simulink model "Approx_Multiplier_M1_AMA1"  (R2021a)
settings: Solver=VariableStepAuto  StartTime=0.0  StopTime=0.01  RelTol=1e-3
(part 2 of 3)

== system Approx_Multiplier_M1_AMA1/Full Adder33 ==
  A : Inport
  B : Inport  Port=2
  Cin : Inport  Port=3
  Half Adder : Subsystem
  Half Adder1 : Subsystem
  Logical Operator : Logic  Operator=OR  AllPortsSameDT=off  OutDataTypeStr=boolean
  Sum : Outport
  Carry : Outport  Port=2
  wires:
  Cin/1 -> Half Adder1/1(In)
  Half Adder1/2(Cout) -> Logical Operator/1
  Half Adder/1(Sum) -> Half Adder1/2(Cin)
  Half Adder1/1(Sum) -> Sum/1
  Half Adder/2(Cout) -> Logical Operator/2
  A/1 -> Half Adder/1(In)
  B/1 -> Half Adder/2(Cin)
  Logical Operator/1 -> Carry/1

== system Approx_Multiplier_M1_AMA1/Full Adder34 ==
  A : Inport
  B : Inport  Port=2
  Cin : Inport  Port=3
  Half Adder : Subsystem
  Half Adder1 : Subsystem
  Logical Operator : Logic  Operator=OR  AllPortsSameDT=off  OutDataTypeStr=boolean
  Sum : Outport
  Carry : Outport  Port=2
  wires:
  Cin/1 -> Half Adder1/1(In)
  Half Adder1/2(Cout) -> Logical Operator/1
  Half Adder/1(Sum) -> Half Adder1/2(Cin)
  Half Adder1/1(Sum) -> Sum/1
  Half Adder/2(Cout) -> Logical Operator/2
  A/1 -> Half Adder/1(In)
  B/1 -> Half Adder/2(Cin)
  Logical Operator/1 -> Carry/1

== system Approx_Multiplier_M1_AMA1/Full Adder36 ==
  A : Inport
  B : Inport  Port=2
  Cin : Inport  Port=3
  Half Adder : Subsystem
  Half Adder1 : Subsystem
  Logical Operator : Logic  Operator=OR  AllPortsSameDT=off  OutDataTypeStr=boolean
  Sum : Outport
  Carry : Outport  Port=2
  wires:
  Cin/1 -> Half Adder1/1(In)
  Half Adder1/2(Cout) -> Logical Operator/1
  Half Adder/1(Sum) -> Half Adder1/2(Cin)
  Half Adder1/1(Sum) -> Sum/1
  Half Adder/2(Cout) -> Logical Operator/2
  A/1 -> Half Adder/1(In)
  B/1 -> Half Adder/2(Cin)
  Logical Operator/1 -> Carry/1

== system Approx_Multiplier_M1_AMA1/Full Adder37 ==
  A : Inport
  B : Inport  Port=2
  Cin : Inport  Port=3
  Half Adder : Subsystem
  Half Adder1 : Subsystem
  Logical Operator : Logic  Operator=OR  AllPortsSameDT=off  OutDataTypeStr=boolean
  Sum : Outport
  Carry : Outport  Port=2
  wires:
  Cin/1 -> Half Adder1/1(In)
  Half Adder1/2(Cout) -> Logical Operator/1
  Half Adder/1(Sum) -> Half Adder1/2(Cin)
  Half Adder1/1(Sum) -> Sum/1
  Half Adder/2(Cout) -> Logical Operator/2
  A/1 -> Half Adder/1(In)
  B/1 -> Half Adder/2(Cin)
  Logical Operator/1 -> Carry/1

== system Approx_Multiplier_M1_AMA1/Full Adder38 ==
  A : Inport
  B : Inport  Port=2
  Cin : Inport  Port=3
  Half Adder : Subsystem
  Half Adder1 : Subsystem
  Logical Operator : Logic  Operator=OR  AllPortsSameDT=off  OutDataTypeStr=boolean
  Sum : Outport
  Carry : Outport  Port=2
  wires:
  Cin/1 -> Half Adder1/1(In)
  Half Adder1/2(Cout) -> Logical Operator/1
  Half Adder/1(Sum) -> Half Adder1/2(Cin)
  Half Adder1/1(Sum) -> Sum/1
  Half Adder/2(Cout) -> Logical Operator/2
  A/1 -> Half Adder/1(In)
  B/1 -> Half Adder/2(Cin)
  Logical Operator/1 -> Carry/1

== system Approx_Multiplier_M1_AMA1/Full Adder39 ==
  A : Inport
  B : Inport  Port=2
  Cin : Inport  Port=3
  Half Adder : Subsystem
  Half Adder1 : Subsystem
  Logical Operator : Logic  Operator=OR  AllPortsSameDT=off  OutDataTypeStr=boolean
  Sum : Outport
  Carry : Outport  Port=2
  wires:
  Cin/1 -> Half Adder1/1(In)
  Half Adder1/2(Cout) -> Logical Operator/1
  Half Adder/1(Sum) -> Half Adder1/2(Cin)
  Half Adder1/1(Sum) -> Sum/1
  Half Adder/2(Cout) -> Logical Operator/2
  A/1 -> Half Adder/1(In)
  B/1 -> Half Adder/2(Cin)
  Logical Operator/1 -> Carry/1

== system Approx_Multiplier_M1_AMA1/Full Adder40 ==
  A : Inport
  B : Inport  Port=2
  Cin : Inport  Port=3
  Half Adder : Subsystem
  Half Adder1 : Subsystem
  Logical Operator : Logic  Operator=OR  AllPortsSameDT=off  OutDataTypeStr=boolean
  Sum : Outport
  Carry : Outport  Port=2
  wires:
  Cin/1 -> Half Adder1/1(In)
  Half Adder1/2(Cout) -> Logical Operator/1
  Half Adder/1(Sum) -> Half Adder1/2(Cin)
  Half Adder1/1(Sum) -> Sum/1
  Half Adder/2(Cout) -> Logical Operator/2
  A/1 -> Half Adder/1(In)
  B/1 -> Half Adder/2(Cin)
  Logical Operator/1 -> Carry/1

== system Approx_Multiplier_M1_AMA1/Full Adder41 ==
  A : Inport
  B : Inport  Port=2
  Cin : Inport  Port=3
  Half Adder : Subsystem
  Half Adder1 : Subsystem
  Logical Operator : Logic  Operator=OR  AllPortsSameDT=off  OutDataTypeStr=boolean
  Sum : Outport
  Carry : Outport  Port=2
  wires:
  Cin/1 -> Half Adder1/1(In)
  Half Adder1/2(Cout) -> Logical Operator/1
  Half Adder/1(Sum) -> Half Adder1/2(Cin)
  Half Adder1/1(Sum) -> Sum/1
  Half Adder/2(Cout) -> Logical Operator/2
  A/1 -> Half Adder/1(In)
  B/1 -> Half Adder/2(Cin)
  Logical Operator/1 -> Carry/1

== system Approx_Multiplier_M1_AMA1/Full Adder42 ==
  A : Inport
  B : Inport  Port=2
  Cin : Inport  Port=3
  Half Adder : Subsystem
  Half Adder1 : Subsystem
  Logical Operator : Logic  Operator=OR  AllPortsSameDT=off  OutDataTypeStr=boolean
  Sum : Outport
  Carry : Outport  Port=2
  wires:
  Cin/1 -> Half Adder1/1(In)
  Half Adder1/2(Cout) -> Logical Operator/1
  Half Adder/1(Sum) -> Half Adder1/2(Cin)
  Half Adder1/1(Sum) -> Sum/1
  Half Adder/2(Cout) -> Logical Operator/2
  A/1 -> Half Adder/1(In)
  B/1 -> Half Adder/2(Cin)
  Logical Operator/1 -> Carry/1

== system Approx_Multiplier_M1_AMA1/Full Adder43 ==
  A : Inport
  B : Inport  Port=2
  Cin : Inport  Port=3
  Half Adder : Subsystem
  Half Adder1 : Subsystem
  Logical Operator : Logic  Operator=OR  AllPortsSameDT=off  OutDataTypeStr=boolean
  Sum : Outport
  Carry : Outport  Port=2
  wires:
  Cin/1 -> Half Adder1/1(In)
  Half Adder1/2(Cout) -> Logical Operator/1
  Half Adder/1(Sum) -> Half Adder1/2(Cin)
  Half Adder1/1(Sum) -> Sum/1
  Half Adder/2(Cout) -> Logical Operator/2
  A/1 -> Half Adder/1(In)
  B/1 -> Half Adder/2(Cin)
  Logical Operator/1 -> Carry/1

== system Approx_Multiplier_M1_AMA1/Full Adder44 ==
  A : Inport
  B : Inport  Port=2
  Cin : Inport  Port=3
  Half Adder : Subsystem
  Half Adder1 : Subsystem
  Logical Operator : Logic  Operator=OR  AllPortsSameDT=off  OutDataTypeStr=boolean
  Sum : Outport
  Carry : Outport  Port=2
  wires:
  Cin/1 -> Half Adder1/1(In)
  Half Adder1/2(Cout) -> Logical Operator/1
  Half Adder/1(Sum) -> Half Adder1/2(Cin)
  Half Adder1/1(Sum) -> Sum/1
  Half Adder/2(Cout) -> Logical Operator/2
  A/1 -> Half Adder/1(In)
  B/1 -> Half Adder/2(Cin)
  Logical Operator/1 -> Carry/1

== system Approx_Multiplier_M1_AMA1/Full Adder45 ==
  A : Inport
  B : Inport  Port=2
  Cin : Inport  Port=3
  Half Adder : Subsystem
  Half Adder1 : Subsystem
  Logical Operator : Logic  Operator=OR  AllPortsSameDT=off  OutDataTypeStr=boolean
  Sum : Outport
  Carry : Outport  Port=2
  wires:
  Cin/1 -> Half Adder1/1(In)
  Half Adder1/2(Cout) -> Logical Operator/1
  Half Adder/1(Sum) -> Half Adder1/2(Cin)
  Half Adder1/1(Sum) -> Sum/1
  Half Adder/2(Cout) -> Logical Operator/2
  A/1 -> Half Adder/1(In)
  B/1 -> Half Adder/2(Cin)
  Logical Operator/1 -> Carry/1

== system Approx_Multiplier_M1_AMA1/Full Adder46 ==
  A : Inport
  B : Inport  Port=2
  Cin : Inport  Port=3
  Half Adder : Subsystem
  Half Adder1 : Subsystem
  Logical Operator : Logic  Operator=OR  AllPortsSameDT=off  OutDataTypeStr=boolean
  Sum : Outport
  Carry : Outport  Port=2
  wires:
  Cin/1 -> Half Adder1/1(In)
  Half Adder1/2(Cout) -> Logical Operator/1
  Half Adder/1(Sum) -> Half Adder1/2(Cin)
  Half Adder1/1(Sum) -> Sum/1
  Half Adder/2(Cout) -> Logical Operator/2
  A/1 -> Half Adder/1(In)
  B/1 -> Half Adder/2(Cin)
  Logical Operator/1 -> Carry/1

== system Approx_Multiplier_M1_AMA1/Full Adder47 ==
  A : Inport
  B : Inport  Port=2
  Cin : Inport  Port=3
  Half Adder : Subsystem
  Half Adder1 : Subsystem
  Logical Operator : Logic  Operator=OR  AllPortsSameDT=off  OutDataTypeStr=boolean
  Sum : Outport
  Carry : Outport  Port=2
  wires:
  Cin/1 -> Half Adder1/1(In)
  Half Adder1/2(Cout) -> Logical Operator/1
  Half Adder/1(Sum) -> Half Adder1/2(Cin)
  Half Adder1/1(Sum) -> Sum/1
  Half Adder/2(Cout) -> Logical Operator/2
  A/1 -> Half Adder/1(In)
  B/1 -> Half Adder/2(Cin)
  Logical Operator/1 -> Carry/1

== system Approx_Multiplier_M1_AMA1/Full Adder48 ==
  A : Inport
  B : Inport  Port=2
  Cin : Inport  Port=3
  Half Adder : Subsystem
  Half Adder1 : Subsystem
  Logical Operator : Logic  Operator=OR  AllPortsSameDT=off  OutDataTypeStr=boolean
  Sum : Outport
  Carry : Outport  Port=2
  wires:
  Cin/1 -> Half Adder1/1(In)
  Half Adder1/2(Cout) -> Logical Operator/1
  Half Adder/1(Sum) -> Half Adder1/2(Cin)
  Half Adder1/1(Sum) -> Sum/1
  Half Adder/2(Cout) -> Logical Operator/2
  A/1 -> Half Adder/1(In)
  B/1 -> Half Adder/2(Cin)
  Logical Operator/1 -> Carry/1

== system Approx_Multiplier_M1_AMA1/Full Adder6 ==
  A : Inport
  B : Inport  Port=2
  Cin : Inport  Port=3
  Half Adder : Subsystem
  Half Adder1 : Subsystem
  Logical Operator : Logic  Operator=OR  AllPortsSameDT=off  OutDataTypeStr=boolean
  Sum : Outport
  Carry : Outport  Port=2
  wires:
  Cin/1 -> Half Adder1/1(In)
  Half Adder1/2(Cout) -> Logical Operator/1
  Half Adder/1(Sum) -> Half Adder1/2(Cin)
  Half Adder1/1(Sum) -> Sum/1
  Half Adder/2(Cout) -> Logical Operator/2
  A/1 -> Half Adder/1(In)
  B/1 -> Half Adder/2(Cin)
  Logical Operator/1 -> Carry/1

== system Approx_Multiplier_M1_AMA1/Half Adder10 ==
  A7B2 : Inport
  Cin : Inport  Port=2
  Logical Operator : Logic  Operator=XOR  AllPortsSameDT=off  OutDataTypeStr=boolean
  Logical Operator1 : Logic  AllPortsSameDT=off  OutDataTypeStr=boolean
  Sum : Outport
  Cout : Outport  Port=2
  wires:
  A7B2/1 -> Logical Operator1/1, Logical Operator/1
  Cin/1 -> Logical Operator/2, Logical Operator1/2
  Logical Operator/1 -> Sum/1
  Logical Operator1/1 -> Cout/1

== system Approx_Multiplier_M1_AMA1/Half Adder11 ==
  A7B2 : Inport
  Cin : Inport  Port=2
  Logical Operator : Logic  Operator=XOR  AllPortsSameDT=off  OutDataTypeStr=boolean
  Logical Operator1 : Logic  AllPortsSameDT=off  OutDataTypeStr=boolean
  Sum : Outport
  Cout : Outport  Port=2
  wires:
  A7B2/1 -> Logical Operator1/1, Logical Operator/1
  Cin/1 -> Logical Operator/2, Logical Operator1/2
  Logical Operator/1 -> Sum/1
  Logical Operator1/1 -> Cout/1

== system Approx_Multiplier_M1_AMA1/Half Adder12 ==
  A7B2 : Inport
  Cin : Inport  Port=2
  Logical Operator : Logic  Operator=XOR  AllPortsSameDT=off  OutDataTypeStr=boolean
  Logical Operator1 : Logic  AllPortsSameDT=off  OutDataTypeStr=boolean
  Sum : Outport
  Cout : Outport  Port=2
  wires:
  A7B2/1 -> Logical Operator1/1, Logical Operator/1
  Cin/1 -> Logical Operator/2, Logical Operator1/2
  Logical Operator/1 -> Sum/1
  Logical Operator1/1 -> Cout/1

== system Approx_Multiplier_M1_AMA1/Half Adder13 ==
  A7B2 : Inport
  Cin : Inport  Port=2
  Logical Operator : Logic  Operator=XOR  AllPortsSameDT=off  OutDataTypeStr=boolean
  Logical Operator1 : Logic  AllPortsSameDT=off  OutDataTypeStr=boolean
  Sum : Outport
  Cout : Outport  Port=2
  wires:
  A7B2/1 -> Logical Operator1/1, Logical Operator/1
  Cin/1 -> Logical Operator/2, Logical Operator1/2
  Logical Operator/1 -> Sum/1
  Logical Operator1/1 -> Cout/1

== system Approx_Multiplier_M1_AMA1/Half Adder7 ==
  Cin : Inport
  Cin1 : Inport  Port=2
  Logical Operator : Logic  Operator=XOR  AllPortsSameDT=off  OutDataTypeStr=boolean
  Logical Operator1 : Logic  AllPortsSameDT=off  OutDataTypeStr=boolean
  Sum : Outport
  Cout : Outport  Port=2
  wires:
  Cin/1 -> Logical Operator1/2, Logical Operator/2
  Logical Operator/1 -> Sum/1
  Logical Operator1/1 -> Cout/1
  Cin1/1 -> Logical Operator1/1, Logical Operator/1

== system Approx_Multiplier_M1_AMA1/Half Adder8 ==
  A7B2 : Inport
  Cin : Inport  Port=2
  Logical Operator : Logic  Operator=XOR  AllPortsSameDT=off  OutDataTypeStr=boolean
  Logical Operator1 : Logic  AllPortsSameDT=off  OutDataTypeStr=boolean
  Sum : Outport
  Cout : Outport  Port=2
  wires:
  A7B2/1 -> Logical Operator1/1, Logical Operator/1
  Cin/1 -> Logical Operator/2, Logical Operator1/2
  Logical Operator/1 -> Sum/1
  Logical Operator1/1 -> Cout/1

== system Approx_Multiplier_M1_AMA1/Half Adder9 ==
  A7B2 : Inport
  Cin : Inport  Port=2
  Logical Operator : Logic  Operator=XOR  AllPortsSameDT=off  OutDataTypeStr=boolean
  Logical Operator1 : Logic  AllPortsSameDT=off  OutDataTypeStr=boolean
  Sum : Outport
  Cout : Outport  Port=2
  wires:
  A7B2/1 -> Logical Operator1/1, Logical Operator/1
  Cin/1 -> Logical Operator/2, Logical Operator1/2
  Logical Operator/1 -> Sum/1
  Logical Operator1/1 -> Cout/1

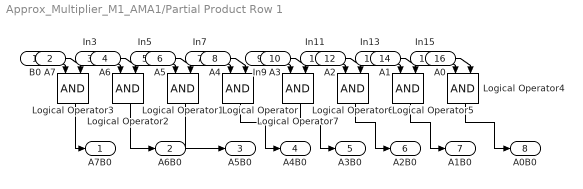
== system Approx_Multiplier_M1_AMA1/Partial Product Row 1 ==
  B0 : Inport
  A7 : Inport  Port=2
  In3 : Inport  Port=3
  A6 : Inport  Port=4
  In5 : Inport  Port=5
  A5 : Inport  Port=6
  In7 : Inport  Port=7
  A4 : Inport  Port=8
  In9 : Inport  Port=9
  A3 : Inport  Port=10
  In11 : Inport  Port=11
  A2 : Inport  Port=12
  In13 : Inport  Port=13
  A1 : Inport  Port=14
  In15 : Inport  Port=15
  A0 : Inport  Port=16
  Logical Operator{,1..7} (8 alike) : Logic  AllPortsSameDT=off  OutDataTypeStr=boolean
  A7B0 : Outport
  A6B0 : Outport  Port=2
  A5B0 : Outport  Port=3
  A4B0 : Outport  Port=4
  A3B0 : Outport  Port=5
  A2B0 : Outport  Port=6
  A1B0 : Outport  Port=7
  A0B0 : Outport  Port=8
  wires:
  Logical Operator7/1 -> A3B0/1
  Logical Operator4/1 -> A0B0/1
  A4/1 -> Logical Operator/2
  Logical Operator/1 -> A4B0/1
  Logical Operator1/1 -> A5B0/1
  A7/1 -> Logical Operator3/2
  In11/1 -> Logical Operator6/1
  In5/1 -> Logical Operator1/1
  A5/1 -> Logical Operator1/2
  In7/1 -> Logical Operator/1
  A6/1 -> Logical Operator2/2
  B0/1 -> Logical Operator3/1
  A2/1 -> Logical Operator6/2
  Logical Operator3/1 -> A7B0/1
  In3/1 -> Logical Operator2/1
  Logical Operator2/1 -> A6B0/1
  In13/1 -> Logical Operator5/1
  A1/1 -> Logical Operator5/2
  Logical Operator5/1 -> A1B0/1
  Logical Operator6/1 -> A2B0/1
  In9/1 -> Logical Operator7/1
  A3/1 -> Logical Operator7/2
  In15/1 -> Logical Operator4/1
  A0/1 -> Logical Operator4/2

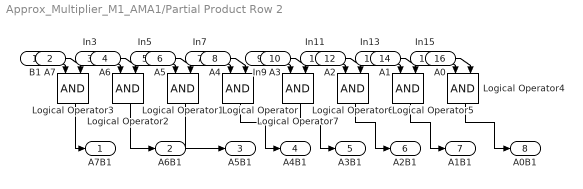
== system Approx_Multiplier_M1_AMA1/Partial Product Row 2 ==
  B1 : Inport
  A7 : Inport  Port=2
  In3 : Inport  Port=3
  A6 : Inport  Port=4
  In5 : Inport  Port=5
  A5 : Inport  Port=6
  In7 : Inport  Port=7
  A4 : Inport  Port=8
  In9 : Inport  Port=9
  A3 : Inport  Port=10
  In11 : Inport  Port=11
  A2 : Inport  Port=12
  In13 : Inport  Port=13
  A1 : Inport  Port=14
  In15 : Inport  Port=15
  A0 : Inport  Port=16
  Logical Operator{,1..7} (8 alike) : Logic  AllPortsSameDT=off  OutDataTypeStr=boolean
  A7B1 : Outport
  A6B1 : Outport  Port=2
  A5B1 : Outport  Port=3
  A4B1 : Outport  Port=4
  A3B1 : Outport  Port=5
  A2B1 : Outport  Port=6
  A1B1 : Outport  Port=7
  A0B1 : Outport  Port=8
  wires:
  Logical Operator7/1 -> A3B1/1
  Logical Operator4/1 -> A0B1/1
  A4/1 -> Logical Operator/2
  Logical Operator/1 -> A4B1/1
  Logical Operator1/1 -> A5B1/1
  A7/1 -> Logical Operator3/2
  In11/1 -> Logical Operator6/1
  In5/1 -> Logical Operator1/1
  A5/1 -> Logical Operator1/2
  In7/1 -> Logical Operator/1
  A6/1 -> Logical Operator2/2
  B1/1 -> Logical Operator3/1
  A2/1 -> Logical Operator6/2
  Logical Operator3/1 -> A7B1/1
  In3/1 -> Logical Operator2/1
  Logical Operator2/1 -> A6B1/1
  In13/1 -> Logical Operator5/1
  A1/1 -> Logical Operator5/2
  Logical Operator5/1 -> A1B1/1
  Logical Operator6/1 -> A2B1/1
  In9/1 -> Logical Operator7/1
  A3/1 -> Logical Operator7/2
  In15/1 -> Logical Operator4/1
  A0/1 -> Logical Operator4/2

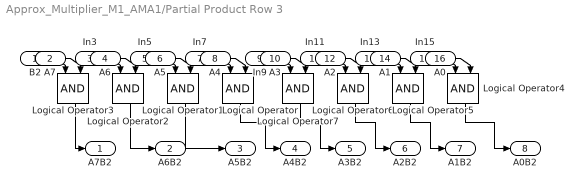
== system Approx_Multiplier_M1_AMA1/Partial Product Row 3 ==
  B2 : Inport
  A7 : Inport  Port=2
  In3 : Inport  Port=3
  A6 : Inport  Port=4
  In5 : Inport  Port=5
  A5 : Inport  Port=6
  In7 : Inport  Port=7
  A4 : Inport  Port=8
  In9 : Inport  Port=9
  A3 : Inport  Port=10
  In11 : Inport  Port=11
  A2 : Inport  Port=12
  In13 : Inport  Port=13
  A1 : Inport  Port=14
  In15 : Inport  Port=15
  A0 : Inport  Port=16
  Logical Operator{,1..7} (8 alike) : Logic  AllPortsSameDT=off  OutDataTypeStr=boolean
  A7B2 : Outport
  A6B2 : Outport  Port=2
  A5B2 : Outport  Port=3
  A4B2 : Outport  Port=4
  A3B2 : Outport  Port=5
  A2B2 : Outport  Port=6
  A1B2 : Outport  Port=7
  A0B2 : Outport  Port=8
  wires:
  Logical Operator7/1 -> A3B2/1
  Logical Operator4/1 -> A0B2/1
  A4/1 -> Logical Operator/2
  Logical Operator/1 -> A4B2/1
  Logical Operator1/1 -> A5B2/1
  A7/1 -> Logical Operator3/2
  In11/1 -> Logical Operator6/1
  In5/1 -> Logical Operator1/1
  A5/1 -> Logical Operator1/2
  In7/1 -> Logical Operator/1
  A6/1 -> Logical Operator2/2
  B2/1 -> Logical Operator3/1
  A2/1 -> Logical Operator6/2
  Logical Operator3/1 -> A7B2/1
  In3/1 -> Logical Operator2/1
  Logical Operator2/1 -> A6B2/1
  In13/1 -> Logical Operator5/1
  A1/1 -> Logical Operator5/2
  Logical Operator5/1 -> A1B2/1
  Logical Operator6/1 -> A2B2/1
  In9/1 -> Logical Operator7/1
  A3/1 -> Logical Operator7/2
  In15/1 -> Logical Operator4/1
  A0/1 -> Logical Operator4/2

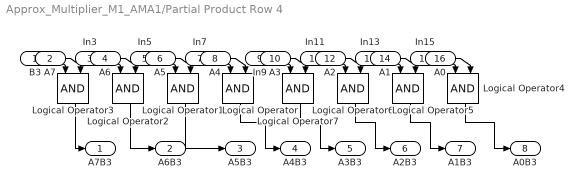
== system Approx_Multiplier_M1_AMA1/Partial Product Row 4 ==
  B3 : Inport
  A7 : Inport  Port=2
  In3 : Inport  Port=3
  A6 : Inport  Port=4
  In5 : Inport  Port=5
  A5 : Inport  Port=6
  In7 : Inport  Port=7
  A4 : Inport  Port=8
  In9 : Inport  Port=9
  A3 : Inport  Port=10
  In11 : Inport  Port=11
  A2 : Inport  Port=12
  In13 : Inport  Port=13
  A1 : Inport  Port=14
  In15 : Inport  Port=15
  A0 : Inport  Port=16
  Logical Operator{,1..7} (8 alike) : Logic  AllPortsSameDT=off  OutDataTypeStr=boolean
  A7B3 : Outport
  A6B3 : Outport  Port=2
  A5B3 : Outport  Port=3
  A4B3 : Outport  Port=4
  A3B3 : Outport  Port=5
  A2B3 : Outport  Port=6
  A1B3 : Outport  Port=7
  A0B3 : Outport  Port=8
  wires:
  Logical Operator7/1 -> A3B3/1
  Logical Operator4/1 -> A0B3/1
  A4/1 -> Logical Operator/2
  Logical Operator/1 -> A4B3/1
  Logical Operator1/1 -> A5B3/1
  A7/1 -> Logical Operator3/2
  In11/1 -> Logical Operator6/1
  In5/1 -> Logical Operator1/1
  A5/1 -> Logical Operator1/2
  In7/1 -> Logical Operator/1
  A6/1 -> Logical Operator2/2
  B3/1 -> Logical Operator3/1
  A2/1 -> Logical Operator6/2
  Logical Operator3/1 -> A7B3/1
  In3/1 -> Logical Operator2/1
  Logical Operator2/1 -> A6B3/1
  In13/1 -> Logical Operator5/1
  A1/1 -> Logical Operator5/2
  Logical Operator5/1 -> A1B3/1
  Logical Operator6/1 -> A2B3/1
  In9/1 -> Logical Operator7/1
  A3/1 -> Logical Operator7/2
  In15/1 -> Logical Operator4/1
  A0/1 -> Logical Operator4/2

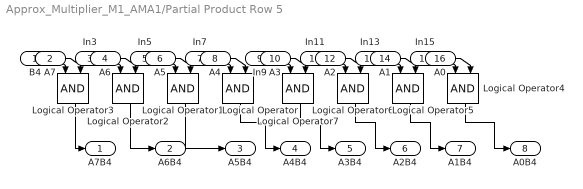
== system Approx_Multiplier_M1_AMA1/Partial Product Row 5 ==
  B4 : Inport
  A7 : Inport  Port=2
  In3 : Inport  Port=3
  A6 : Inport  Port=4
  In5 : Inport  Port=5
  A5 : Inport  Port=6
  In7 : Inport  Port=7
  A4 : Inport  Port=8
  In9 : Inport  Port=9
  A3 : Inport  Port=10
  In11 : Inport  Port=11
  A2 : Inport  Port=12
  In13 : Inport  Port=13
  A1 : Inport  Port=14
  In15 : Inport  Port=15
  A0 : Inport  Port=16
  Logical Operator{,1..7} (8 alike) : Logic  AllPortsSameDT=off  OutDataTypeStr=boolean
  A7B4 : Outport
  A6B4 : Outport  Port=2
  A5B4 : Outport  Port=3
  A4B4 : Outport  Port=4
  A3B4 : Outport  Port=5
  A2B4 : Outport  Port=6
  A1B4 : Outport  Port=7
  A0B4 : Outport  Port=8
  wires:
  Logical Operator7/1 -> A3B4/1
  Logical Operator4/1 -> A0B4/1
  A4/1 -> Logical Operator/2
  Logical Operator/1 -> A4B4/1
  Logical Operator1/1 -> A5B4/1
  A7/1 -> Logical Operator3/2
  In11/1 -> Logical Operator6/1
  In5/1 -> Logical Operator1/1
  A5/1 -> Logical Operator1/2
  In7/1 -> Logical Operator/1
  A6/1 -> Logical Operator2/2
  B4/1 -> Logical Operator3/1
  A2/1 -> Logical Operator6/2
  Logical Operator3/1 -> A7B4/1
  In3/1 -> Logical Operator2/1
  Logical Operator2/1 -> A6B4/1
  In13/1 -> Logical Operator5/1
  A1/1 -> Logical Operator5/2
  Logical Operator5/1 -> A1B4/1
  Logical Operator6/1 -> A2B4/1
  In9/1 -> Logical Operator7/1
  A3/1 -> Logical Operator7/2
  In15/1 -> Logical Operator4/1
  A0/1 -> Logical Operator4/2

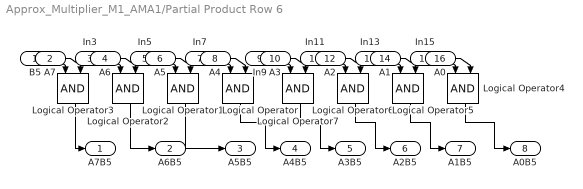
== system Approx_Multiplier_M1_AMA1/Partial Product Row 6 ==
  B5 : Inport
  A7 : Inport  Port=2
  In3 : Inport  Port=3
  A6 : Inport  Port=4
  In5 : Inport  Port=5
  A5 : Inport  Port=6
  In7 : Inport  Port=7
  A4 : Inport  Port=8
  In9 : Inport  Port=9
  A3 : Inport  Port=10
  In11 : Inport  Port=11
  A2 : Inport  Port=12
  In13 : Inport  Port=13
  A1 : Inport  Port=14
  In15 : Inport  Port=15
  A0 : Inport  Port=16
  Logical Operator{,1..7} (8 alike) : Logic  AllPortsSameDT=off  OutDataTypeStr=boolean
  A7B5 : Outport
  A6B5 : Outport  Port=2
  A5B5 : Outport  Port=3
  A4B5 : Outport  Port=4
  A3B5 : Outport  Port=5
  A2B5 : Outport  Port=6
  A1B5 : Outport  Port=7
  A0B5 : Outport  Port=8
  wires:
  Logical Operator7/1 -> A3B5/1
  Logical Operator4/1 -> A0B5/1
  A4/1 -> Logical Operator/2
  Logical Operator/1 -> A4B5/1
  Logical Operator1/1 -> A5B5/1
  A7/1 -> Logical Operator3/2
  In11/1 -> Logical Operator6/1
  In5/1 -> Logical Operator1/1
  A5/1 -> Logical Operator1/2
  In7/1 -> Logical Operator/1
  A6/1 -> Logical Operator2/2
  B5/1 -> Logical Operator3/1
  A2/1 -> Logical Operator6/2
  Logical Operator3/1 -> A7B5/1
  In3/1 -> Logical Operator2/1
  Logical Operator2/1 -> A6B5/1
  In13/1 -> Logical Operator5/1
  A1/1 -> Logical Operator5/2
  Logical Operator5/1 -> A1B5/1
  Logical Operator6/1 -> A2B5/1
  In9/1 -> Logical Operator7/1
  A3/1 -> Logical Operator7/2
  In15/1 -> Logical Operator4/1
  A0/1 -> Logical Operator4/2

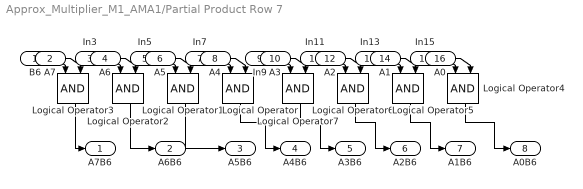
== system Approx_Multiplier_M1_AMA1/Partial Product Row 7 ==
  B6 : Inport
  A7 : Inport  Port=2
  In3 : Inport  Port=3
  A6 : Inport  Port=4
  In5 : Inport  Port=5
  A5 : Inport  Port=6
  In7 : Inport  Port=7
  A4 : Inport  Port=8
  In9 : Inport  Port=9
  A3 : Inport  Port=10
  In11 : Inport  Port=11
  A2 : Inport  Port=12
  In13 : Inport  Port=13
  A1 : Inport  Port=14
  In15 : Inport  Port=15
  A0 : Inport  Port=16
  Logical Operator{,1..7} (8 alike) : Logic  AllPortsSameDT=off  OutDataTypeStr=boolean
  A7B6 : Outport
  A6B6 : Outport  Port=2
  A5B6 : Outport  Port=3
  A4B6 : Outport  Port=4
  A3B6 : Outport  Port=5
  A2B6 : Outport  Port=6
  A1B6 : Outport  Port=7
  A0B6 : Outport  Port=8
  wires:
  Logical Operator7/1 -> A3B6/1
  Logical Operator4/1 -> A0B6/1
  A4/1 -> Logical Operator/2
  Logical Operator/1 -> A4B6/1
  Logical Operator1/1 -> A5B6/1
  A7/1 -> Logical Operator3/2
  In11/1 -> Logical Operator6/1
  In5/1 -> Logical Operator1/1
  A5/1 -> Logical Operator1/2
  In7/1 -> Logical Operator/1
  A6/1 -> Logical Operator2/2
  B6/1 -> Logical Operator3/1
  A2/1 -> Logical Operator6/2
  Logical Operator3/1 -> A7B6/1
  In3/1 -> Logical Operator2/1
  Logical Operator2/1 -> A6B6/1
  In13/1 -> Logical Operator5/1
  A1/1 -> Logical Operator5/2
  Logical Operator5/1 -> A1B6/1
  Logical Operator6/1 -> A2B6/1
  In9/1 -> Logical Operator7/1
  A3/1 -> Logical Operator7/2
  In15/1 -> Logical Operator4/1
  A0/1 -> Logical Operator4/2

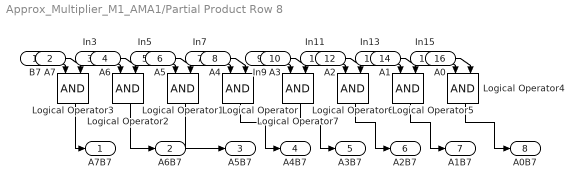
== system Approx_Multiplier_M1_AMA1/Partial Product Row 8 ==
  B7 : Inport
  A7 : Inport  Port=2
  In3 : Inport  Port=3
  A6 : Inport  Port=4
  In5 : Inport  Port=5
  A5 : Inport  Port=6
  In7 : Inport  Port=7
  A4 : Inport  Port=8
  In9 : Inport  Port=9
  A3 : Inport  Port=10
  In11 : Inport  Port=11
  A2 : Inport  Port=12
  In13 : Inport  Port=13
  A1 : Inport  Port=14
  In15 : Inport  Port=15
  A0 : Inport  Port=16
  Logical Operator{,1..7} (8 alike) : Logic  AllPortsSameDT=off  OutDataTypeStr=boolean
  A7B7 : Outport
  A6B7 : Outport  Port=2
  A5B7 : Outport  Port=3
  A4B7 : Outport  Port=4
  A3B7 : Outport  Port=5
  A2B7 : Outport  Port=6
  A1B7 : Outport  Port=7
  A0B7 : Outport  Port=8
  wires:
  Logical Operator7/1 -> A3B7/1
  Logical Operator4/1 -> A0B7/1
  A4/1 -> Logical Operator/2
  Logical Operator/1 -> A4B7/1
  Logical Operator1/1 -> A5B7/1
  A7/1 -> Logical Operator3/2
  In11/1 -> Logical Operator6/1
  In5/1 -> Logical Operator1/1
  A5/1 -> Logical Operator1/2
  In7/1 -> Logical Operator/1
  A6/1 -> Logical Operator2/2
  B7/1 -> Logical Operator3/1
  A2/1 -> Logical Operator6/2
  Logical Operator3/1 -> A7B7/1
  In3/1 -> Logical Operator2/1
  Logical Operator2/1 -> A6B7/1
  In13/1 -> Logical Operator5/1
  A1/1 -> Logical Operator5/2
  Logical Operator5/1 -> A1B7/1
  Logical Operator6/1 -> A2B7/1
  In9/1 -> Logical Operator7/1
  A3/1 -> Logical Operator7/2
  In15/1 -> Logical Operator4/1
  A0/1 -> Logical Operator4/2

== system Approx_Multiplier_M1_AMA1/Full Adder12/Half Adder ==
  In : Inport
  Cin : Inport  Port=2
  Logical Operator : Logic  Operator=XOR  AllPortsSameDT=off  OutDataTypeStr=boolean
  Logical Operator1 : Logic  AllPortsSameDT=off  OutDataTypeStr=boolean
  Sum : Outport
  Cout : Outport  Port=2
  wires:
  In/1 -> Logical Operator1/1, Logical Operator/1
  Cin/1 -> Logical Operator/2, Logical Operator1/2
  Logical Operator/1 -> Sum/1
  Logical Operator1/1 -> Cout/1

== system Approx_Multiplier_M1_AMA1/Full Adder12/Half Adder1 ==
  In : Inport
  Cin : Inport  Port=2
  Logical Operator : Logic  Operator=XOR  AllPortsSameDT=off  OutDataTypeStr=boolean
  Logical Operator1 : Logic  AllPortsSameDT=off  OutDataTypeStr=boolean
  Sum : Outport
  Cout : Outport  Port=2
  wires:
  In/1 -> Logical Operator1/1, Logical Operator/1
  Cin/1 -> Logical Operator/2, Logical Operator1/2
  Logical Operator/1 -> Sum/1
  Logical Operator1/1 -> Cout/1

== system Approx_Multiplier_M1_AMA1/Full Adder13/Half Adder ==
  In : Inport
  Cin : Inport  Port=2
  Logical Operator : Logic  Operator=XOR  AllPortsSameDT=off  OutDataTypeStr=boolean
  Logical Operator1 : Logic  AllPortsSameDT=off  OutDataTypeStr=boolean
  Sum : Outport
  Cout : Outport  Port=2
  wires:
  In/1 -> Logical Operator1/1, Logical Operator/1
  Cin/1 -> Logical Operator/2, Logical Operator1/2
  Logical Operator/1 -> Sum/1
  Logical Operator1/1 -> Cout/1

== system Approx_Multiplier_M1_AMA1/Full Adder13/Half Adder1 ==
  In : Inport
  Cin : Inport  Port=2
  Logical Operator : Logic  Operator=XOR  AllPortsSameDT=off  OutDataTypeStr=boolean
  Logical Operator1 : Logic  AllPortsSameDT=off  OutDataTypeStr=boolean
  Sum : Outport
  Cout : Outport  Port=2
  wires:
  In/1 -> Logical Operator1/1, Logical Operator/1
  Cin/1 -> Logical Operator/2, Logical Operator1/2
  Logical Operator/1 -> Sum/1
  Logical Operator1/1 -> Cout/1

== system Approx_Multiplier_M1_AMA1/Full Adder18/Half Adder ==
  In : Inport
  Cin : Inport  Port=2
  Logical Operator : Logic  Operator=XOR  AllPortsSameDT=off  OutDataTypeStr=boolean
  Logical Operator1 : Logic  AllPortsSameDT=off  OutDataTypeStr=boolean
  Sum : Outport
  Cout : Outport  Port=2
  wires:
  In/1 -> Logical Operator1/1, Logical Operator/1
  Cin/1 -> Logical Operator/2, Logical Operator1/2
  Logical Operator/1 -> Sum/1
  Logical Operator1/1 -> Cout/1

== system Approx_Multiplier_M1_AMA1/Full Adder18/Half Adder1 ==
  In : Inport
  Cin : Inport  Port=2
  Logical Operator : Logic  Operator=XOR  AllPortsSameDT=off  OutDataTypeStr=boolean
  Logical Operator1 : Logic  AllPortsSameDT=off  OutDataTypeStr=boolean
  Sum : Outport
  Cout : Outport  Port=2
  wires:
  In/1 -> Logical Operator1/1, Logical Operator/1
  Cin/1 -> Logical Operator/2, Logical Operator1/2
  Logical Operator/1 -> Sum/1
  Logical Operator1/1 -> Cout/1

== system Approx_Multiplier_M1_AMA1/Full Adder19/Half Adder ==
  In : Inport
  Cin : Inport  Port=2
  Logical Operator : Logic  Operator=XOR  AllPortsSameDT=off  OutDataTypeStr=boolean
  Logical Operator1 : Logic  AllPortsSameDT=off  OutDataTypeStr=boolean
  Sum : Outport
  Cout : Outport  Port=2
  wires:
  In/1 -> Logical Operator1/1, Logical Operator/1
  Cin/1 -> Logical Operator/2, Logical Operator1/2
  Logical Operator/1 -> Sum/1
  Logical Operator1/1 -> Cout/1

== system Approx_Multiplier_M1_AMA1/Full Adder19/Half Adder1 ==
  In : Inport
  Cin : Inport  Port=2
  Logical Operator : Logic  Operator=XOR  AllPortsSameDT=off  OutDataTypeStr=boolean
  Logical Operator1 : Logic  AllPortsSameDT=off  OutDataTypeStr=boolean
  Sum : Outport
  Cout : Outport  Port=2
  wires:
  In/1 -> Logical Operator1/1, Logical Operator/1
  Cin/1 -> Logical Operator/2, Logical Operator1/2
  Logical Operator/1 -> Sum/1
  Logical Operator1/1 -> Cout/1

== system Approx_Multiplier_M1_AMA1/Full Adder20/Half Adder ==
  In : Inport
  Cin : Inport  Port=2
  Logical Operator : Logic  Operator=XOR  AllPortsSameDT=off  OutDataTypeStr=boolean
  Logical Operator1 : Logic  AllPortsSameDT=off  OutDataTypeStr=boolean
  Sum : Outport
  Cout : Outport  Port=2
  wires:
  In/1 -> Logical Operator1/1, Logical Operator/1
  Cin/1 -> Logical Operator/2, Logical Operator1/2
  Logical Operator/1 -> Sum/1
  Logical Operator1/1 -> Cout/1

== system Approx_Multiplier_M1_AMA1/Full Adder20/Half Adder1 ==
  In : Inport
  Cin : Inport  Port=2
  Logical Operator : Logic  Operator=XOR  AllPortsSameDT=off  OutDataTypeStr=boolean
  Logical Operator1 : Logic  AllPortsSameDT=off  OutDataTypeStr=boolean
  Sum : Outport
  Cout : Outport  Port=2
  wires:
  In/1 -> Logical Operator1/1, Logical Operator/1
  Cin/1 -> Logical Operator/2, Logical Operator1/2
  Logical Operator/1 -> Sum/1
  Logical Operator1/1 -> Cout/1

== system Approx_Multiplier_M1_AMA1/Full Adder24/Half Adder ==
  In : Inport
  Cin : Inport  Port=2
  Logical Operator : Logic  Operator=XOR  AllPortsSameDT=off  OutDataTypeStr=boolean
  Logical Operator1 : Logic  AllPortsSameDT=off  OutDataTypeStr=boolean
  Sum : Outport
  Cout : Outport  Port=2
  wires:
  In/1 -> Logical Operator1/1, Logical Operator/1
  Cin/1 -> Logical Operator/2, Logical Operator1/2
  Logical Operator/1 -> Sum/1
  Logical Operator1/1 -> Cout/1

== system Approx_Multiplier_M1_AMA1/Full Adder24/Half Adder1 ==
  In : Inport
  Cin : Inport  Port=2
  Logical Operator : Logic  Operator=XOR  AllPortsSameDT=off  OutDataTypeStr=boolean
  Logical Operator1 : Logic  AllPortsSameDT=off  OutDataTypeStr=boolean
  Sum : Outport
  Cout : Outport  Port=2
  wires:
  In/1 -> Logical Operator1/1, Logical Operator/1
  Cin/1 -> Logical Operator/2, Logical Operator1/2
  Logical Operator/1 -> Sum/1
  Logical Operator1/1 -> Cout/1

== system Approx_Multiplier_M1_AMA1/Full Adder25/Half Adder ==
  In : Inport
  Cin : Inport  Port=2
  Logical Operator : Logic  Operator=XOR  AllPortsSameDT=off  OutDataTypeStr=boolean
  Logical Operator1 : Logic  AllPortsSameDT=off  OutDataTypeStr=boolean
  Sum : Outport
  Cout : Outport  Port=2
  wires:
  In/1 -> Logical Operator1/1, Logical Operator/1
  Cin/1 -> Logical Operator/2, Logical Operator1/2
  Logical Operator/1 -> Sum/1
  Logical Operator1/1 -> Cout/1

== system Approx_Multiplier_M1_AMA1/Full Adder25/Half Adder1 ==
  In : Inport
  Cin : Inport  Port=2
  Logical Operator : Logic  Operator=XOR  AllPortsSameDT=off  OutDataTypeStr=boolean
  Logical Operator1 : Logic  AllPortsSameDT=off  OutDataTypeStr=boolean
  Sum : Outport
  Cout : Outport  Port=2
  wires:
  In/1 -> Logical Operator1/1, Logical Operator/1
  Cin/1 -> Logical Operator/2, Logical Operator1/2
  Logical Operator/1 -> Sum/1
  Logical Operator1/1 -> Cout/1

== system Approx_Multiplier_M1_AMA1/Full Adder26/Half Adder ==
  In : Inport
  Cin : Inport  Port=2
  Logical Operator : Logic  Operator=XOR  AllPortsSameDT=off  OutDataTypeStr=boolean
  Logical Operator1 : Logic  AllPortsSameDT=off  OutDataTypeStr=boolean
  Sum : Outport
  Cout : Outport  Port=2
  wires:
  In/1 -> Logical Operator1/1, Logical Operator/1
  Cin/1 -> Logical Operator/2, Logical Operator1/2
  Logical Operator/1 -> Sum/1
  Logical Operator1/1 -> Cout/1

== system Approx_Multiplier_M1_AMA1/Full Adder26/Half Adder1 ==
  In : Inport
  Cin : Inport  Port=2
  Logical Operator : Logic  Operator=XOR  AllPortsSameDT=off  OutDataTypeStr=boolean
  Logical Operator1 : Logic  AllPortsSameDT=off  OutDataTypeStr=boolean
  Sum : Outport
  Cout : Outport  Port=2
  wires:
  In/1 -> Logical Operator1/1, Logical Operator/1
  Cin/1 -> Logical Operator/2, Logical Operator1/2
  Logical Operator/1 -> Sum/1
  Logical Operator1/1 -> Cout/1

== system Approx_Multiplier_M1_AMA1/Full Adder27/Half Adder ==
  In : Inport
  Cin : Inport  Port=2
  Logical Operator : Logic  Operator=XOR  AllPortsSameDT=off  OutDataTypeStr=boolean
  Logical Operator1 : Logic  AllPortsSameDT=off  OutDataTypeStr=boolean
  Sum : Outport
  Cout : Outport  Port=2
  wires:
  In/1 -> Logical Operator1/1, Logical Operator/1
  Cin/1 -> Logical Operator/2, Logical Operator1/2
  Logical Operator/1 -> Sum/1
  Logical Operator1/1 -> Cout/1

== system Approx_Multiplier_M1_AMA1/Full Adder27/Half Adder1 ==
  In : Inport
  Cin : Inport  Port=2
  Logical Operator : Logic  Operator=XOR  AllPortsSameDT=off  OutDataTypeStr=boolean
  Logical Operator1 : Logic  AllPortsSameDT=off  OutDataTypeStr=boolean
  Sum : Outport
  Cout : Outport  Port=2
  wires:
  In/1 -> Logical Operator1/1, Logical Operator/1
  Cin/1 -> Logical Operator/2, Logical Operator1/2
  Logical Operator/1 -> Sum/1
  Logical Operator1/1 -> Cout/1

== system Approx_Multiplier_M1_AMA1/Full Adder30/Half Adder ==
  In : Inport
  Cin : Inport  Port=2
  Logical Operator : Logic  Operator=XOR  AllPortsSameDT=off  OutDataTypeStr=boolean
  Logical Operator1 : Logic  AllPortsSameDT=off  OutDataTypeStr=boolean
  Sum : Outport
  Cout : Outport  Port=2
  wires:
  In/1 -> Logical Operator1/1, Logical Operator/1
  Cin/1 -> Logical Operator/2, Logical Operator1/2
  Logical Operator/1 -> Sum/1
  Logical Operator1/1 -> Cout/1

== system Approx_Multiplier_M1_AMA1/Full Adder30/Half Adder1 ==
  In : Inport
  Cin : Inport  Port=2
  Logical Operator : Logic  Operator=XOR  AllPortsSameDT=off  OutDataTypeStr=boolean
  Logical Operator1 : Logic  AllPortsSameDT=off  OutDataTypeStr=boolean
  Sum : Outport
  Cout : Outport  Port=2
  wires:
  In/1 -> Logical Operator1/1, Logical Operator/1
  Cin/1 -> Logical Operator/2, Logical Operator1/2
  Logical Operator/1 -> Sum/1
  Logical Operator1/1 -> Cout/1

== system Approx_Multiplier_M1_AMA1/Full Adder31/Half Adder ==
  In : Inport
  Cin : Inport  Port=2
  Logical Operator : Logic  Operator=XOR  AllPortsSameDT=off  OutDataTypeStr=boolean
  Logical Operator1 : Logic  AllPortsSameDT=off  OutDataTypeStr=boolean
  Sum : Outport
  Cout : Outport  Port=2
  wires:
  In/1 -> Logical Operator1/1, Logical Operator/1
  Cin/1 -> Logical Operator/2, Logical Operator1/2
  Logical Operator/1 -> Sum/1
  Logical Operator1/1 -> Cout/1

== system Approx_Multiplier_M1_AMA1/Full Adder31/Half Adder1 ==
  In : Inport
  Cin : Inport  Port=2
  Logical Operator : Logic  Operator=XOR  AllPortsSameDT=off  OutDataTypeStr=boolean
  Logical Operator1 : Logic  AllPortsSameDT=off  OutDataTypeStr=boolean
  Sum : Outport
  Cout : Outport  Port=2
  wires:
  In/1 -> Logical Operator1/1, Logical Operator/1
  Cin/1 -> Logical Operator/2, Logical Operator1/2
  Logical Operator/1 -> Sum/1
  Logical Operator1/1 -> Cout/1

== system Approx_Multiplier_M1_AMA1/Full Adder32/Half Adder ==
  In : Inport
  Cin : Inport  Port=2
  Logical Operator : Logic  Operator=XOR  AllPortsSameDT=off  OutDataTypeStr=boolean
  Logical Operator1 : Logic  AllPortsSameDT=off  OutDataTypeStr=boolean
  Sum : Outport
  Cout : Outport  Port=2
  wires:
  In/1 -> Logical Operator1/1, Logical Operator/1
  Cin/1 -> Logical Operator/2, Logical Operator1/2
  Logical Operator/1 -> Sum/1
  Logical Operator1/1 -> Cout/1

== system Approx_Multiplier_M1_AMA1/Full Adder32/Half Adder1 ==
  In : Inport
  Cin : Inport  Port=2
  Logical Operator : Logic  Operator=XOR  AllPortsSameDT=off  OutDataTypeStr=boolean
  Logical Operator1 : Logic  AllPortsSameDT=off  OutDataTypeStr=boolean
  Sum : Outport
  Cout : Outport  Port=2
  wires:
  In/1 -> Logical Operator1/1, Logical Operator/1
  Cin/1 -> Logical Operator/2, Logical Operator1/2
  Logical Operator/1 -> Sum/1
  Logical Operator1/1 -> Cout/1

== system Approx_Multiplier_M1_AMA1/Full Adder33/Half Adder ==
  In : Inport
  Cin : Inport  Port=2
  Logical Operator : Logic  Operator=XOR  AllPortsSameDT=off  OutDataTypeStr=boolean
  Logical Operator1 : Logic  AllPortsSameDT=off  OutDataTypeStr=boolean
  Sum : Outport
  Cout : Outport  Port=2
  wires:
  In/1 -> Logical Operator1/1, Logical Operator/1
  Cin/1 -> Logical Operator/2, Logical Operator1/2
  Logical Operator/1 -> Sum/1
  Logical Operator1/1 -> Cout/1

== system Approx_Multiplier_M1_AMA1/Full Adder33/Half Adder1 ==
  In : Inport
  Cin : Inport  Port=2
  Logical Operator : Logic  Operator=XOR  AllPortsSameDT=off  OutDataTypeStr=boolean
  Logical Operator1 : Logic  AllPortsSameDT=off  OutDataTypeStr=boolean
  Sum : Outport
  Cout : Outport  Port=2
  wires:
  In/1 -> Logical Operator1/1, Logical Operator/1
  Cin/1 -> Logical Operator/2, Logical Operator1/2
  Logical Operator/1 -> Sum/1
  Logical Operator1/1 -> Cout/1

== system Approx_Multiplier_M1_AMA1/Full Adder34/Half Adder ==
  In : Inport
  Cin : Inport  Port=2
  Logical Operator : Logic  Operator=XOR  AllPortsSameDT=off  OutDataTypeStr=boolean
  Logical Operator1 : Logic  AllPortsSameDT=off  OutDataTypeStr=boolean
  Sum : Outport
  Cout : Outport  Port=2
  wires:
  In/1 -> Logical Operator1/1, Logical Operator/1
  Cin/1 -> Logical Operator/2, Logical Operator1/2
  Logical Operator/1 -> Sum/1
  Logical Operator1/1 -> Cout/1

== system Approx_Multiplier_M1_AMA1/Full Adder34/Half Adder1 ==
  In : Inport
  Cin : Inport  Port=2
  Logical Operator : Logic  Operator=XOR  AllPortsSameDT=off  OutDataTypeStr=boolean
  Logical Operator1 : Logic  AllPortsSameDT=off  OutDataTypeStr=boolean
  Sum : Outport
  Cout : Outport  Port=2
  wires:
  In/1 -> Logical Operator1/1, Logical Operator/1
  Cin/1 -> Logical Operator/2, Logical Operator1/2
  Logical Operator/1 -> Sum/1
  Logical Operator1/1 -> Cout/1

== system Approx_Multiplier_M1_AMA1/Full Adder36/Half Adder ==
  In : Inport
  Cin : Inport  Port=2
  Logical Operator : Logic  Operator=XOR  AllPortsSameDT=off  OutDataTypeStr=boolean
  Logical Operator1 : Logic  AllPortsSameDT=off  OutDataTypeStr=boolean
  Sum : Outport
  Cout : Outport  Port=2
  wires:
  In/1 -> Logical Operator1/1, Logical Operator/1
  Cin/1 -> Logical Operator/2, Logical Operator1/2
  Logical Operator/1 -> Sum/1
  Logical Operator1/1 -> Cout/1

== system Approx_Multiplier_M1_AMA1/Full Adder36/Half Adder1 ==
  In : Inport
  Cin : Inport  Port=2
  Logical Operator : Logic  Operator=XOR  AllPortsSameDT=off  OutDataTypeStr=boolean
  Logical Operator1 : Logic  AllPortsSameDT=off  OutDataTypeStr=boolean
  Sum : Outport
  Cout : Outport  Port=2
  wires:
  In/1 -> Logical Operator1/1, Logical Operator/1
  Cin/1 -> Logical Operator/2, Logical Operator1/2
  Logical Operator/1 -> Sum/1
  Logical Operator1/1 -> Cout/1

== system Approx_Multiplier_M1_AMA1/Full Adder37/Half Adder ==
  In : Inport
  Cin : Inport  Port=2
  Logical Operator : Logic  Operator=XOR  AllPortsSameDT=off  OutDataTypeStr=boolean
  Logical Operator1 : Logic  AllPortsSameDT=off  OutDataTypeStr=boolean
  Sum : Outport
  Cout : Outport  Port=2
  wires:
  In/1 -> Logical Operator1/1, Logical Operator/1
  Cin/1 -> Logical Operator/2, Logical Operator1/2
  Logical Operator/1 -> Sum/1
  Logical Operator1/1 -> Cout/1

== system Approx_Multiplier_M1_AMA1/Full Adder37/Half Adder1 ==
  In : Inport
  Cin : Inport  Port=2
  Logical Operator : Logic  Operator=XOR  AllPortsSameDT=off  OutDataTypeStr=boolean
  Logical Operator1 : Logic  AllPortsSameDT=off  OutDataTypeStr=boolean
  Sum : Outport
  Cout : Outport  Port=2
  wires:
  In/1 -> Logical Operator1/1, Logical Operator/1
  Cin/1 -> Logical Operator/2, Logical Operator1/2
  Logical Operator/1 -> Sum/1
  Logical Operator1/1 -> Cout/1

== system Approx_Multiplier_M1_AMA1/Full Adder38/Half Adder ==
  In : Inport
  Cin : Inport  Port=2
  Logical Operator : Logic  Operator=XOR  AllPortsSameDT=off  OutDataTypeStr=boolean
  Logical Operator1 : Logic  AllPortsSameDT=off  OutDataTypeStr=boolean
  Sum : Outport
  Cout : Outport  Port=2
  wires:
  In/1 -> Logical Operator1/1, Logical Operator/1
  Cin/1 -> Logical Operator/2, Logical Operator1/2
  Logical Operator/1 -> Sum/1
  Logical Operator1/1 -> Cout/1

== system Approx_Multiplier_M1_AMA1/Full Adder38/Half Adder1 ==
  In : Inport
  Cin : Inport  Port=2
  Logical Operator : Logic  Operator=XOR  AllPortsSameDT=off  OutDataTypeStr=boolean
  Logical Operator1 : Logic  AllPortsSameDT=off  OutDataTypeStr=boolean
  Sum : Outport
  Cout : Outport  Port=2
  wires:
  In/1 -> Logical Operator1/1, Logical Operator/1
  Cin/1 -> Logical Operator/2, Logical Operator1/2
  Logical Operator/1 -> Sum/1
  Logical Operator1/1 -> Cout/1

== system Approx_Multiplier_M1_AMA1/Full Adder39/Half Adder ==
  In : Inport
  Cin : Inport  Port=2
  Logical Operator : Logic  Operator=XOR  AllPortsSameDT=off  OutDataTypeStr=boolean
  Logical Operator1 : Logic  AllPortsSameDT=off  OutDataTypeStr=boolean
  Sum : Outport
  Cout : Outport  Port=2
  wires:
  In/1 -> Logical Operator1/1, Logical Operator/1
  Cin/1 -> Logical Operator/2, Logical Operator1/2
  Logical Operator/1 -> Sum/1
  Logical Operator1/1 -> Cout/1

== system Approx_Multiplier_M1_AMA1/Full Adder39/Half Adder1 ==
  In : Inport
  Cin : Inport  Port=2
  Logical Operator : Logic  Operator=XOR  AllPortsSameDT=off  OutDataTypeStr=boolean
  Logical Operator1 : Logic  AllPortsSameDT=off  OutDataTypeStr=boolean
  Sum : Outport
  Cout : Outport  Port=2
  wires:
  In/1 -> Logical Operator1/1, Logical Operator/1
  Cin/1 -> Logical Operator/2, Logical Operator1/2
  Logical Operator/1 -> Sum/1
  Logical Operator1/1 -> Cout/1

== system Approx_Multiplier_M1_AMA1/Full Adder40/Half Adder ==
  In : Inport
  Cin : Inport  Port=2
  Logical Operator : Logic  Operator=XOR  AllPortsSameDT=off  OutDataTypeStr=boolean
  Logical Operator1 : Logic  AllPortsSameDT=off  OutDataTypeStr=boolean
  Sum : Outport
  Cout : Outport  Port=2
  wires:
  In/1 -> Logical Operator1/1, Logical Operator/1
  Cin/1 -> Logical Operator/2, Logical Operator1/2
  Logical Operator/1 -> Sum/1
  Logical Operator1/1 -> Cout/1

== system Approx_Multiplier_M1_AMA1/Full Adder40/Half Adder1 ==
  In : Inport
  Cin : Inport  Port=2
  Logical Operator : Logic  Operator=XOR  AllPortsSameDT=off  OutDataTypeStr=boolean
  Logical Operator1 : Logic  AllPortsSameDT=off  OutDataTypeStr=boolean
  Sum : Outport
  Cout : Outport  Port=2
  wires:
  In/1 -> Logical Operator1/1, Logical Operator/1
  Cin/1 -> Logical Operator/2, Logical Operator1/2
  Logical Operator/1 -> Sum/1
  Logical Operator1/1 -> Cout/1

== system Approx_Multiplier_M1_AMA1/Full Adder41/Half Adder ==
  In : Inport
  Cin : Inport  Port=2
  Logical Operator : Logic  Operator=XOR  AllPortsSameDT=off  OutDataTypeStr=boolean
  Logical Operator1 : Logic  AllPortsSameDT=off  OutDataTypeStr=boolean
  Sum : Outport
  Cout : Outport  Port=2
  wires:
  In/1 -> Logical Operator1/1, Logical Operator/1
  Cin/1 -> Logical Operator/2, Logical Operator1/2
  Logical Operator/1 -> Sum/1
  Logical Operator1/1 -> Cout/1

== system Approx_Multiplier_M1_AMA1/Full Adder41/Half Adder1 ==
  In : Inport
  Cin : Inport  Port=2
  Logical Operator : Logic  Operator=XOR  AllPortsSameDT=off  OutDataTypeStr=boolean
  Logical Operator1 : Logic  AllPortsSameDT=off  OutDataTypeStr=boolean
  Sum : Outport
  Cout : Outport  Port=2
  wires:
  In/1 -> Logical Operator1/1, Logical Operator/1
  Cin/1 -> Logical Operator/2, Logical Operator1/2
  Logical Operator/1 -> Sum/1
  Logical Operator1/1 -> Cout/1

== system Approx_Multiplier_M1_AMA1/Full Adder42/Half Adder ==
  In : Inport
  Cin : Inport  Port=2
  Logical Operator : Logic  Operator=XOR  AllPortsSameDT=off  OutDataTypeStr=boolean
  Logical Operator1 : Logic  AllPortsSameDT=off  OutDataTypeStr=boolean
  Sum : Outport
  Cout : Outport  Port=2
  wires:
  In/1 -> Logical Operator1/1, Logical Operator/1
  Cin/1 -> Logical Operator/2, Logical Operator1/2
  Logical Operator/1 -> Sum/1
  Logical Operator1/1 -> Cout/1

== system Approx_Multiplier_M1_AMA1/Full Adder42/Half Adder1 ==
  In : Inport
  Cin : Inport  Port=2
  Logical Operator : Logic  Operator=XOR  AllPortsSameDT=off  OutDataTypeStr=boolean
  Logical Operator1 : Logic  AllPortsSameDT=off  OutDataTypeStr=boolean
  Sum : Outport
  Cout : Outport  Port=2
  wires:
  In/1 -> Logical Operator1/1, Logical Operator/1
  Cin/1 -> Logical Operator/2, Logical Operator1/2
  Logical Operator/1 -> Sum/1
  Logical Operator1/1 -> Cout/1

== system Approx_Multiplier_M1_AMA1/Full Adder43/Half Adder ==
  In : Inport
  Cin : Inport  Port=2
  Logical Operator : Logic  Operator=XOR  AllPortsSameDT=off  OutDataTypeStr=boolean
  Logical Operator1 : Logic  AllPortsSameDT=off  OutDataTypeStr=boolean
  Sum : Outport
  Cout : Outport  Port=2
  wires:
  In/1 -> Logical Operator1/1, Logical Operator/1
  Cin/1 -> Logical Operator/2, Logical Operator1/2
  Logical Operator/1 -> Sum/1
  Logical Operator1/1 -> Cout/1

== system Approx_Multiplier_M1_AMA1/Full Adder43/Half Adder1 ==
  In : Inport
  Cin : Inport  Port=2
  Logical Operator : Logic  Operator=XOR  AllPortsSameDT=off  OutDataTypeStr=boolean
  Logical Operator1 : Logic  AllPortsSameDT=off  OutDataTypeStr=boolean
  Sum : Outport
  Cout : Outport  Port=2
  wires:
  In/1 -> Logical Operator1/1, Logical Operator/1
  Cin/1 -> Logical Operator/2, Logical Operator1/2
  Logical Operator/1 -> Sum/1
  Logical Operator1/1 -> Cout/1

== system Approx_Multiplier_M1_AMA1/Full Adder44/Half Adder ==
  In : Inport
  Cin : Inport  Port=2
  Logical Operator : Logic  Operator=XOR  AllPortsSameDT=off  OutDataTypeStr=boolean
  Logical Operator1 : Logic  AllPortsSameDT=off  OutDataTypeStr=boolean
  Sum : Outport
  Cout : Outport  Port=2
  wires:
  In/1 -> Logical Operator1/1, Logical Operator/1
  Cin/1 -> Logical Operator/2, Logical Operator1/2
  Logical Operator/1 -> Sum/1
  Logical Operator1/1 -> Cout/1

== system Approx_Multiplier_M1_AMA1/Full Adder44/Half Adder1 ==
  In : Inport
  Cin : Inport  Port=2
  Logical Operator : Logic  Operator=XOR  AllPortsSameDT=off  OutDataTypeStr=boolean
  Logical Operator1 : Logic  AllPortsSameDT=off  OutDataTypeStr=boolean
  Sum : Outport
  Cout : Outport  Port=2
  wires:
  In/1 -> Logical Operator1/1, Logical Operator/1
  Cin/1 -> Logical Operator/2, Logical Operator1/2
  Logical Operator/1 -> Sum/1
  Logical Operator1/1 -> Cout/1

== system Approx_Multiplier_M1_AMA1/Full Adder45/Half Adder ==
  In : Inport
  Cin : Inport  Port=2
  Logical Operator : Logic  Operator=XOR  AllPortsSameDT=off  OutDataTypeStr=boolean
  Logical Operator1 : Logic  AllPortsSameDT=off  OutDataTypeStr=boolean
  Sum : Outport
  Cout : Outport  Port=2
  wires:
  In/1 -> Logical Operator1/1, Logical Operator/1
  Cin/1 -> Logical Operator/2, Logical Operator1/2
  Logical Operator/1 -> Sum/1
  Logical Operator1/1 -> Cout/1

== system Approx_Multiplier_M1_AMA1/Full Adder45/Half Adder1 ==
  In : Inport
  Cin : Inport  Port=2
  Logical Operator : Logic  Operator=XOR  AllPortsSameDT=off  OutDataTypeStr=boolean
  Logical Operator1 : Logic  AllPortsSameDT=off  OutDataTypeStr=boolean
  Sum : Outport
  Cout : Outport  Port=2
  wires:
  In/1 -> Logical Operator1/1, Logical Operator/1
  Cin/1 -> Logical Operator/2, Logical Operator1/2
  Logical Operator/1 -> Sum/1
  Logical Operator1/1 -> Cout/1

== system Approx_Multiplier_M1_AMA1/Full Adder46/Half Adder ==
  In : Inport
  Cin : Inport  Port=2
  Logical Operator : Logic  Operator=XOR  AllPortsSameDT=off  OutDataTypeStr=boolean
  Logical Operator1 : Logic  AllPortsSameDT=off  OutDataTypeStr=boolean
  Sum : Outport
  Cout : Outport  Port=2
  wires:
  In/1 -> Logical Operator1/1, Logical Operator/1
  Cin/1 -> Logical Operator/2, Logical Operator1/2
  Logical Operator/1 -> Sum/1
  Logical Operator1/1 -> Cout/1

== system Approx_Multiplier_M1_AMA1/Full Adder46/Half Adder1 ==
  In : Inport
  Cin : Inport  Port=2
  Logical Operator : Logic  Operator=XOR  AllPortsSameDT=off  OutDataTypeStr=boolean
  Logical Operator1 : Logic  AllPortsSameDT=off  OutDataTypeStr=boolean
  Sum : Outport
  Cout : Outport  Port=2
  wires:
  In/1 -> Logical Operator1/1, Logical Operator/1
  Cin/1 -> Logical Operator/2, Logical Operator1/2
  Logical Operator/1 -> Sum/1
  Logical Operator1/1 -> Cout/1

== system Approx_Multiplier_M1_AMA1/Full Adder47/Half Adder ==
  In : Inport
  Cin : Inport  Port=2
  Logical Operator : Logic  Operator=XOR  AllPortsSameDT=off  OutDataTypeStr=boolean
  Logical Operator1 : Logic  AllPortsSameDT=off  OutDataTypeStr=boolean
  Sum : Outport
  Cout : Outport  Port=2
  wires:
  In/1 -> Logical Operator1/1, Logical Operator/1
  Cin/1 -> Logical Operator/2, Logical Operator1/2
  Logical Operator/1 -> Sum/1
  Logical Operator1/1 -> Cout/1

== system Approx_Multiplier_M1_AMA1/Full Adder47/Half Adder1 ==
  In : Inport
  Cin : Inport  Port=2
  Logical Operator : Logic  Operator=XOR  AllPortsSameDT=off  OutDataTypeStr=boolean
  Logical Operator1 : Logic  AllPortsSameDT=off  OutDataTypeStr=boolean
  Sum : Outport
  Cout : Outport  Port=2
  wires:
  In/1 -> Logical Operator1/1, Logical Operator/1
  Cin/1 -> Logical Operator/2, Logical Operator1/2
  Logical Operator/1 -> Sum/1
  Logical Operator1/1 -> Cout/1

== system Approx_Multiplier_M1_AMA1/Full Adder48/Half Adder ==
  In : Inport
  Cin : Inport  Port=2
  Logical Operator : Logic  Operator=XOR  AllPortsSameDT=off  OutDataTypeStr=boolean
  Logical Operator1 : Logic  AllPortsSameDT=off  OutDataTypeStr=boolean
  Sum : Outport
  Cout : Outport  Port=2
  wires:
  In/1 -> Logical Operator1/1, Logical Operator/1
  Cin/1 -> Logical Operator/2, Logical Operator1/2
  Logical Operator/1 -> Sum/1
  Logical Operator1/1 -> Cout/1

== system Approx_Multiplier_M1_AMA1/Full Adder48/Half Adder1 ==
  In : Inport
  Cin : Inport  Port=2
  Logical Operator : Logic  Operator=XOR  AllPortsSameDT=off  OutDataTypeStr=boolean
  Logical Operator1 : Logic  AllPortsSameDT=off  OutDataTypeStr=boolean
  Sum : Outport
  Cout : Outport  Port=2
  wires:
  In/1 -> Logical Operator1/1, Logical Operator/1
  Cin/1 -> Logical Operator/2, Logical Operator1/2
  Logical Operator/1 -> Sum/1
  Logical Operator1/1 -> Cout/1
